simulink model "PWM"  (R2019b)
settings: Solver=VariableStepAuto  StartTime=0.0  StopTime=10.0  FixedStep=1/(PWM_Resolution*PWM_Frequency)  RelTol=1e-3
PreLoadFcn:
  | modelDir = fileparts(get_param(bdroot, 'FileName'));
  | addpath(fullfile(modelDir,'../../Parameters'));
  | 
  | Parameters_Model
  | Parameters_Simulation
  | Parameters_Controller
InitFcn:
  | Parameters_Model
  | Parameters_Simulation
  | Parameters_Controller
undefined symbols (not defined in the file): PWM_Frequency, PWM_Resolution
libraries: simulink x1
settings Model: Creator=Thomas  LastModifiedBy=thomas.jespersen
settings DataIOCC: ReturnWorkspaceOutputs=off
settings DebuggingCC: ArithmeticOperatorsInVariantConditions=warning
settings SFSimCC: SimUseLocalCustomCode=off  CustomCodeUndefinedFunction=UseInterfaceOnly
settings RTWCC: RTWUseLocalCustomCode=off

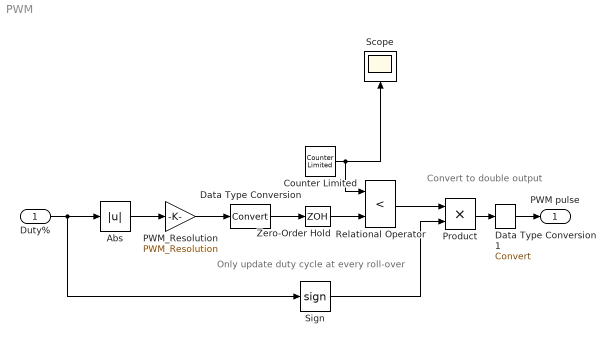
== system PWM ==
  note: Convert to double output
  note: Only update duty cycle at every roll-over
  Duty% : Inport  OutDataTypeStr=double
  Abs : Abs
  Counter Limited : simulink/Sources/Counter Limited  uplimit=PWM_Resolution-1  tsamp=1/(PWM_Resolution*PWM_Frequency)
  Data Type Conversion : DataTypeConversion  RndMeth=Round
  Data Type Conversion1 : DataTypeConversion  RndMeth=Round
  PWM_Resolution : Gain  Gain=PWM_Resolution
  Product : Product
  Relational Operator : RelationalOperator  Operator=<  OutDataTypeStr=boolean  RndMeth=Simplest
  Scope : Scope
  Sign : Signum
  Zero-Order Hold : ZeroOrderHold  SampleTime=1/PWM_Frequency
  PWM pulse : Outport  OutDataTypeStr=int8  VectorParamsAs1DForOutWhenUnconnected=off
  wires:
  Counter Limited/1 -> Scope/1, Relational Operator/1
  Duty%/1 -> Abs/1, Sign/1
  PWM_Resolution/1 -> Data Type Conversion/1
  Zero-Order Hold/1 -> Relational Operator/2
  Data Type Conversion/1 -> Zero-Order Hold/1
  Relational Operator/1 -> Product/1
  Product/1 -> Data Type Conversion1/1
  Sign/1 -> Product/2
  Abs/1 -> PWM_Resolution/1
  Data Type Conversion1/1 -> PWM pulse/1
